simulink model "FRA231_EXAM_1_Y_ID_Y_ID_Y_ID_Y_ID"  (R2020b)
settings: Solver=VariableStepAuto  StartTime=0.0  StopTime=inf  RelTol=1e-3
settings Model: EnablePacing=on  Creator=kittithamrongaphichartkul  LastModifiedBy=TinnP137
settings DebuggingCC: SFMachineParentedDataDiag=error

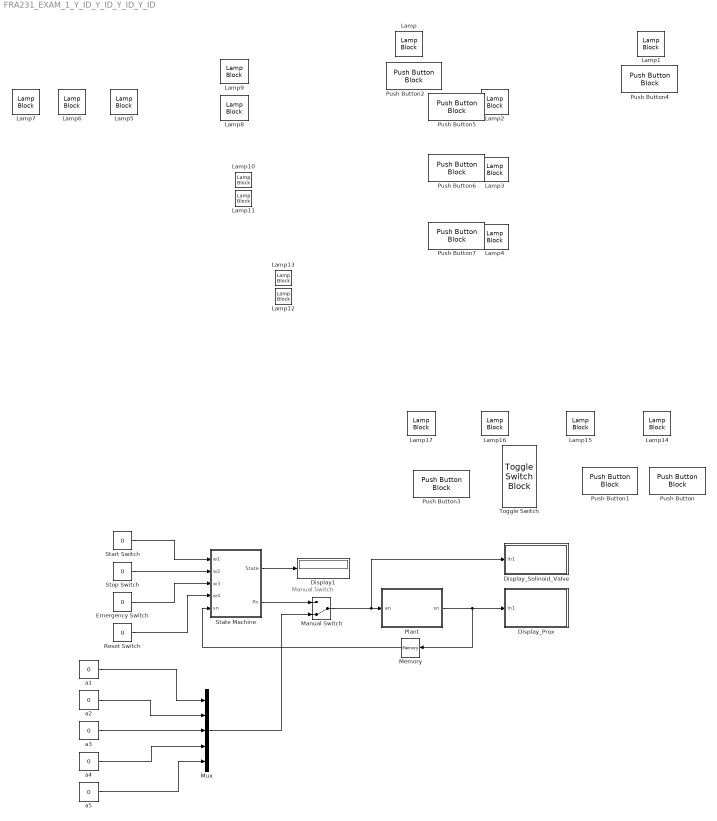
== system FRA231_EXAM_1_Y_ID_Y_ID_Y_ID_Y_ID ==
  note: Manual Switch
  Display1 : Display
  Display_Prox : Subsystem
  Display_Solinoid_Valve : Subsystem
  Emergency Switch : Constant  Value=0  OutDataTypeStr=boolean
  Lamp{,1..17} (18 alike) : LampBlock
  Manual Switch : ManualSwitch  CurrentSetting=0
  Memory : Memory
  Mux : Mux  Inputs=5
  Plant : Subsystem
  Push Button : PushButtonBlock  ButtonText=Start
  Push Button1 : PushButtonBlock  ButtonText=Stop
  Push Button2 : PushButtonBlock  ButtonText=a1
  Push Button3 : PushButtonBlock  ButtonText=Reset
  Push Button4 : PushButtonBlock  ButtonText=a2
  Push Button5 : PushButtonBlock  ButtonText=a3
  Push Button6 : PushButtonBlock  ButtonText=a4
  Push Button7 : PushButtonBlock  ButtonText=a5
  Reset Switch : Constant  Value=0  OutDataTypeStr=boolean
  Start Switch : Constant  Value=0  OutDataTypeStr=boolean
  State Machine : Subsystem
  Stop Switch : Constant  Value=0  OutDataTypeStr=boolean
  Toggle Switch : ToggleSwitchBlock
      settings: Values={{'Off', 'On'}, [0 1]}
  a{1..5} (5 alike) : Constant  Value=0  OutDataTypeStr=boolean
  wires:
  Plant/1(sn) -> Display_Prox/1(In1), Memory/1
  Manual Switch/1 -> Display_Solinoid_Valve/1(In1), Plant/1(an)
  State Machine/2(Pn) -> Manual Switch/1
  Start Switch/1 -> State Machine/1(w1)
  Stop Switch/1 -> State Machine/2(w2)
  Emergency Switch/1 -> State Machine/3(w3)
  Memory/1 -> State Machine/5(sn)
  State Machine/1(State) -> Display1/1
  Reset Switch/1 -> State Machine/4(w4)
  Mux/1 -> Manual Switch/2
  a1/1 -> Mux/1
  a2/1 -> Mux/2
  a3/1 -> Mux/3
  a4/1 -> Mux/4
  a5/1 -> Mux/5

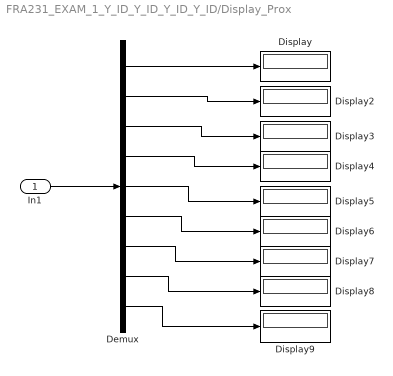
== system FRA231_EXAM_1_Y_ID_Y_ID_Y_ID_Y_ID/Display_Prox ==
  In1 : Inport
  Demux : Demux  Outputs=9
  Display{,2..9} (9 alike) : Display
  wires:
  In1/1 -> Demux/1
  Demux/6 -> Display6/1
  Demux/5 -> Display5/1
  Demux/9 -> Display9/1
  Demux/2 -> Display2/1
  Demux/7 -> Display7/1
  Demux/4 -> Display4/1
  Demux/8 -> Display8/1
  Demux/3 -> Display3/1
  Demux/1 -> Display/1

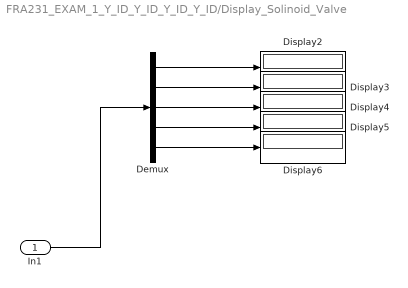
== system FRA231_EXAM_1_Y_ID_Y_ID_Y_ID_Y_ID/Display_Solinoid_Valve ==
  In1 : Inport
  Demux : Demux  Outputs=5
  Display{2..6} (5 alike) : Display
  wires:
  In1/1 -> Demux/1
  Demux/1 -> Display2/1
  Demux/3 -> Display4/1
  Demux/5 -> Display6/1
  Demux/4 -> Display5/1
  Demux/2 -> Display3/1

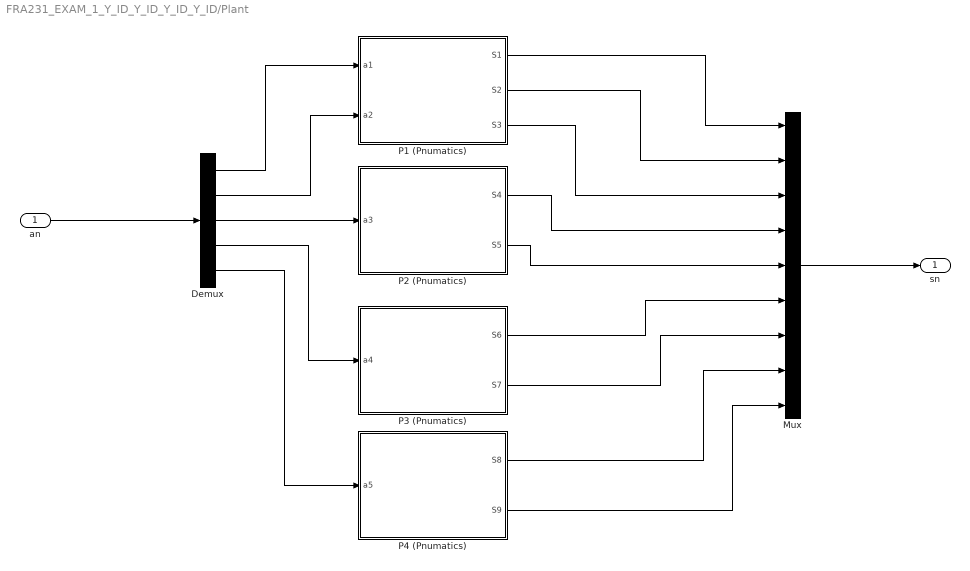
== system FRA231_EXAM_1_Y_ID_Y_ID_Y_ID_Y_ID/Plant ==
  an : Inport
  Demux : Demux  Outputs=5
  Mux : Mux  Inputs=9
  P1 (Pnumatics) : Subsystem
  P2 (Pnumatics) : Subsystem
  P3 (Pnumatics) : Subsystem
  P4 (Pnumatics) : Subsystem
  sn : Outport
  wires:
  an/1 -> Demux/1
  Demux/2 -> P1 (Pnumatics)/2(a2)
  P3 (Pnumatics)/1(S6) -> Mux/6
  P4 (Pnumatics)/2(S9) -> Mux/9
  P1 (Pnumatics)/1(S1) -> Mux/1
  P3 (Pnumatics)/2(S7) -> Mux/7
  Demux/3 -> P2 (Pnumatics)/1(a3)
  P2 (Pnumatics)/1(S4) -> Mux/4
  Mux/1 -> sn/1
  Demux/1 -> P1 (Pnumatics)/1(a1)
  Demux/5 -> P4 (Pnumatics)/1(a5)
  P1 (Pnumatics)/3(S3) -> Mux/3
  Demux/4 -> P3 (Pnumatics)/1(a4)
  P1 (Pnumatics)/2(S2) -> Mux/2
  P4 (Pnumatics)/1(S8) -> Mux/8
  P2 (Pnumatics)/2(S5) -> Mux/5

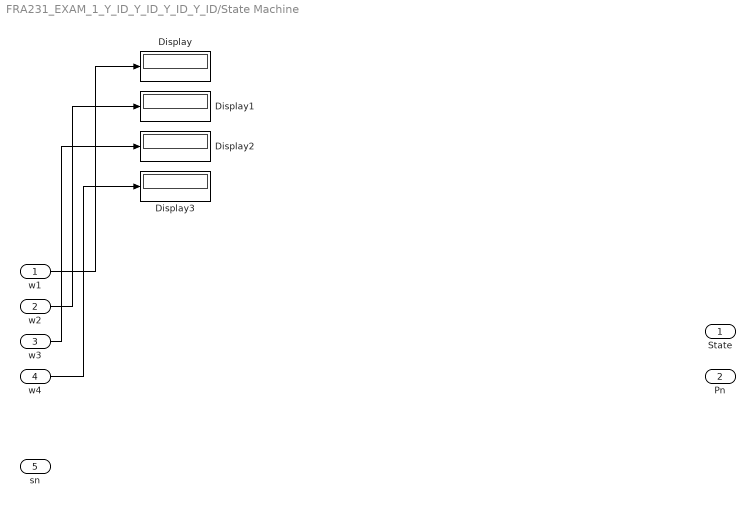
== system FRA231_EXAM_1_Y_ID_Y_ID_Y_ID_Y_ID/State Machine ==
  w1 : Inport
  w2 : Inport  Port=2
  w3 : Inport  Port=3
  w4 : Inport  Port=4
  sn : Inport  Port=5
  Display{,1..3} (4 alike) : Display
  State : Outport
  Pn : Outport  Port=2
  wires:
  w1/1 -> Display/1
  w2/1 -> Display1/1
  w3/1 -> Display2/1
  w4/1 -> Display3/1

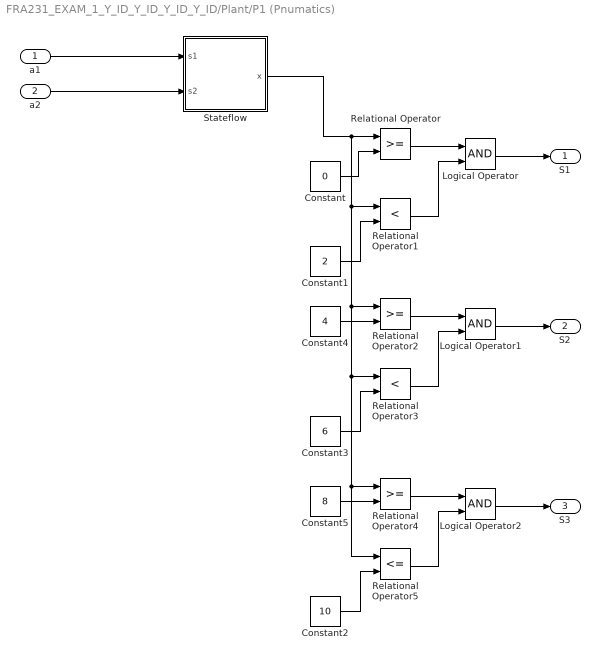
== system FRA231_EXAM_1_Y_ID_Y_ID_Y_ID_Y_ID/Plant/P1 (Pnumatics) ==
  a1 : Inport
  a2 : Inport  Port=2
  Constant : Constant  Value=0
  Constant1 : Constant  Value=2
  Constant2 : Constant  Value=10
  Constant3 : Constant  Value=6
  Constant4 : Constant  Value=4
  Constant5 : Constant  Value=8
  Logical Operator : Logic  AllPortsSameDT=off  OutDataTypeStr=boolean
  Logical Operator1 : Logic  AllPortsSameDT=off  OutDataTypeStr=boolean
  Logical Operator2 : Logic  AllPortsSameDT=off  OutDataTypeStr=boolean
  Relational Operator : RelationalOperator  OutDataTypeStr=boolean  RndMeth=Simplest
  Relational Operator1 : RelationalOperator  Operator=<  OutDataTypeStr=boolean  RndMeth=Simplest
  Relational Operator2 : RelationalOperator  OutDataTypeStr=boolean  RndMeth=Simplest
  Relational Operator3 : RelationalOperator  Operator=<  OutDataTypeStr=boolean  RndMeth=Simplest
  Relational Operator4 : RelationalOperator  OutDataTypeStr=boolean  RndMeth=Simplest
  Relational Operator5 : RelationalOperator  Operator=<=  OutDataTypeStr=boolean  RndMeth=Simplest
  Stateflow : Stateflow chart  AncestorBlock=RoboticsPlayground/Utilities and Hardware/Stateflow  TreatAsAtomicUnit=on
  S1 : Outport
  S2 : Outport  Port=2
  S3 : Outport  Port=3
  wires:
  a1/1 -> Stateflow/1(s1)
  a2/1 -> Stateflow/2(s2)
  Constant/1 -> Relational Operator/2
  Relational Operator/1 -> Logical Operator/1
  Relational Operator1/1 -> Logical Operator/2
  Logical Operator/1 -> S1/1
  Relational Operator2/1 -> Logical Operator1/1
  Constant1/1 -> Relational Operator1/2
  Relational Operator3/1 -> Logical Operator1/2
  Logical Operator1/1 -> S2/1
  Relational Operator5/1 -> Logical Operator2/2
  Relational Operator4/1 -> Logical Operator2/1
  Stateflow/1(x) -> Relational Operator2/1, Relational Operator4/1, Relational Operator5/1, Relational Operator3/1, Relational Operator1/1, Relational Operator/1
  Constant3/1 -> Relational Operator3/2
  Constant2/1 -> Relational Operator5/2
  Logical Operator2/1 -> S3/1
  Constant4/1 -> Relational Operator2/2
  Constant5/1 -> Relational Operator4/2

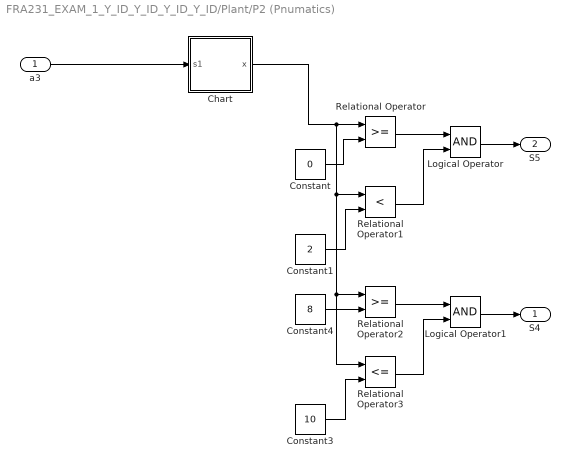
== system FRA231_EXAM_1_Y_ID_Y_ID_Y_ID_Y_ID/Plant/P2 (Pnumatics) ==
  a3 : Inport
  Chart : Stateflow chart  TreatAsAtomicUnit=on
  Constant : Constant  Value=0
  Constant1 : Constant  Value=2
  Constant3 : Constant  Value=10
  Constant4 : Constant  Value=8
  Logical Operator : Logic  AllPortsSameDT=off  OutDataTypeStr=boolean
  Logical Operator1 : Logic  AllPortsSameDT=off  OutDataTypeStr=boolean
  Relational Operator : RelationalOperator  OutDataTypeStr=boolean  RndMeth=Simplest
  Relational Operator1 : RelationalOperator  Operator=<  OutDataTypeStr=boolean  RndMeth=Simplest
  Relational Operator2 : RelationalOperator  OutDataTypeStr=boolean  RndMeth=Simplest
  Relational Operator3 : RelationalOperator  Operator=<=  OutDataTypeStr=boolean  RndMeth=Simplest
  S4 : Outport
  S5 : Outport  Port=2
  wires:
  a3/1 -> Chart/1(s1)
  Chart/1(x) -> Relational Operator2/1, Relational Operator3/1, Relational Operator1/1, Relational Operator/1
  Relational Operator1/1 -> Logical Operator/2
  Constant3/1 -> Relational Operator3/2
  Constant1/1 -> Relational Operator1/2
  Relational Operator/1 -> Logical Operator/1
  Constant/1 -> Relational Operator/2
  Relational Operator3/1 -> Logical Operator1/2
  Relational Operator2/1 -> Logical Operator1/1
  Constant4/1 -> Relational Operator2/2
  Logical Operator1/1 -> S4/1
  Logical Operator/1 -> S5/1

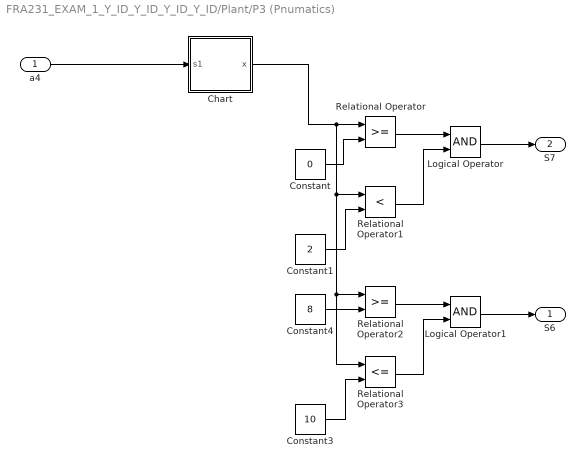
== system FRA231_EXAM_1_Y_ID_Y_ID_Y_ID_Y_ID/Plant/P3 (Pnumatics) ==
  a4 : Inport
  Chart : Stateflow chart  TreatAsAtomicUnit=on
  Constant : Constant  Value=0
  Constant1 : Constant  Value=2
  Constant3 : Constant  Value=10
  Constant4 : Constant  Value=8
  Logical Operator : Logic  AllPortsSameDT=off  OutDataTypeStr=boolean
  Logical Operator1 : Logic  AllPortsSameDT=off  OutDataTypeStr=boolean
  Relational Operator : RelationalOperator  OutDataTypeStr=boolean  RndMeth=Simplest
  Relational Operator1 : RelationalOperator  Operator=<  OutDataTypeStr=boolean  RndMeth=Simplest
  Relational Operator2 : RelationalOperator  OutDataTypeStr=boolean  RndMeth=Simplest
  Relational Operator3 : RelationalOperator  Operator=<=  OutDataTypeStr=boolean  RndMeth=Simplest
  S6 : Outport
  S7 : Outport  Port=2
  wires:
  a4/1 -> Chart/1(s1)
  Chart/1(x) -> Relational Operator2/1, Relational Operator3/1, Relational Operator1/1, Relational Operator/1
  Relational Operator1/1 -> Logical Operator/2
  Constant3/1 -> Relational Operator3/2
  Constant1/1 -> Relational Operator1/2
  Relational Operator/1 -> Logical Operator/1
  Constant/1 -> Relational Operator/2
  Relational Operator3/1 -> Logical Operator1/2
  Relational Operator2/1 -> Logical Operator1/1
  Constant4/1 -> Relational Operator2/2
  Logical Operator/1 -> S7/1
  Logical Operator1/1 -> S6/1

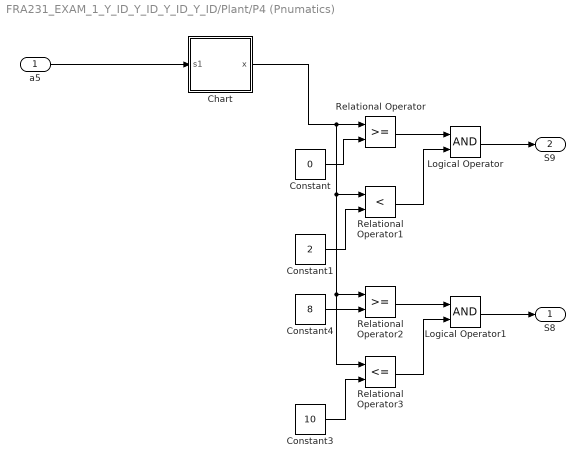
== system FRA231_EXAM_1_Y_ID_Y_ID_Y_ID_Y_ID/Plant/P4 (Pnumatics) ==
  a5 : Inport
  Chart : Stateflow chart  TreatAsAtomicUnit=on
  Constant : Constant  Value=0
  Constant1 : Constant  Value=2
  Constant3 : Constant  Value=10
  Constant4 : Constant  Value=8
  Logical Operator : Logic  AllPortsSameDT=off  OutDataTypeStr=boolean
  Logical Operator1 : Logic  AllPortsSameDT=off  OutDataTypeStr=boolean
  Relational Operator : RelationalOperator  OutDataTypeStr=boolean  RndMeth=Simplest
  Relational Operator1 : RelationalOperator  Operator=<  OutDataTypeStr=boolean  RndMeth=Simplest
  Relational Operator2 : RelationalOperator  OutDataTypeStr=boolean  RndMeth=Simplest
  Relational Operator3 : RelationalOperator  Operator=<=  OutDataTypeStr=boolean  RndMeth=Simplest
  S8 : Outport
  S9 : Outport  Port=2
  wires:
  a5/1 -> Chart/1(s1)
  Chart/1(x) -> Relational Operator2/1, Relational Operator3/1, Relational Operator1/1, Relational Operator/1
  Relational Operator1/1 -> Logical Operator/2
  Constant3/1 -> Relational Operator3/2
  Constant1/1 -> Relational Operator1/2
  Relational Operator/1 -> Logical Operator/1
  Constant/1 -> Relational Operator/2
  Relational Operator3/1 -> Logical Operator1/2
  Relational Operator2/1 -> Logical Operator1/1
  Constant4/1 -> Relational Operator2/2
  Logical Operator1/1 -> S8/1
  Logical Operator/1 -> S9/1

== stateflow chart FRA231_EXAM_1_Y_ID_Y_ID_Y_ID_Y_ID/Plant/P2 (Pnumatics)/Chart ==
  state idel
  state s1
    if x >= x_max
    x = x_max
    else
    x=x + 1;
    end
  state s2
    if x <= x_min
    x = x_min
    else
    x=x - 1;
    end
  (default) -> idel : {
      | x=0,
      | x_max = 10,
      | x_min = 0
      | }
  idel -> s1 [order 2] : [s1==1]
  idel -> s2 [order 1] : [s1==0]
  s1 -> s2 : [s1==0]
  s2 -> s1 : [s1==1]
  data: x output; s1 input; x_min local; x_max local

== stateflow chart FRA231_EXAM_1_Y_ID_Y_ID_Y_ID_Y_ID/Plant/P3 (Pnumatics)/Chart ==
  state idel
  state s1
    if x >= x_max
    x = x_max
    else
    x=x + 1;
    end
  state s2
    if x <= x_min
    x = x_min
    else
    x=x - 1;
    end
  (default) -> idel : {
      | x=0,
      | x_max = 10,
      | x_min = 0
      | }
  idel -> s1 [order 2] : [s1==1]
  idel -> s2 [order 1] : [s1==0]
  s1 -> s2 : [s1==0]
  s2 -> s1 : [s1==1]
  data: x output; s1 input; x_min local; x_max local

== stateflow chart FRA231_EXAM_1_Y_ID_Y_ID_Y_ID_Y_ID/Plant/P1 (Pnumatics)/Stateflow ==
  state idel
  state s1
    if x >= x_max
    x = x_max
    else
    x=x + 1;
    end
  state s2
    if x <= x_min
    x = x_min
    else
    x=x - 1;
    end
  (default) -> idel : {
      | x=0,
      | x_max = 10,
      | x_min = 0
      | }
  idel -> s1 [order 1] : [s1==1 && s2==0]
  idel -> s2 [order 2] : [s1==0&&s2==1]
  s1 -> idel [order 2] : [(s1==0&&s2==0) || (s1==1&&s2==1)]
  s2 -> idel : [(s1==0&&s2==0) || (s1==1&&s2==1)]
  s1 -> s2 [order 1] : [s1==0&&s2==1]
  data: x output; s1 input; StateflowMode local Enum: StateflowModeType; s2 input; x_min local; x_max local

== stateflow chart FRA231_EXAM_1_Y_ID_Y_ID_Y_ID_Y_ID/Plant/P4 (Pnumatics)/Chart ==
  state idel
  state s1
    if x >= x_max
    x = x_max
    else
    x=x + 1;
    end
  state s2
    if x <= x_min
    x = x_min
    else
    x=x - 1;
    end
  (default) -> idel : {
      | x=0,
      | x_max = 10,
      | x_min = 0
      | }
  idel -> s1 [order 2] : [s1==1]
  idel -> s2 [order 1] : [s1==0]
  s1 -> s2 : [s1==0]
  s2 -> s1 : [s1==1]
  data: x output; s1 input; x_min local; x_max local
